simulink model "Counter_condition"  (R2022b)
settings: Solver=VariableStepAuto  StartTime=0.0  StopTime=10.0  RelTol=1e-3
settings Model: Creator=USER  LastModifiedBy=USER

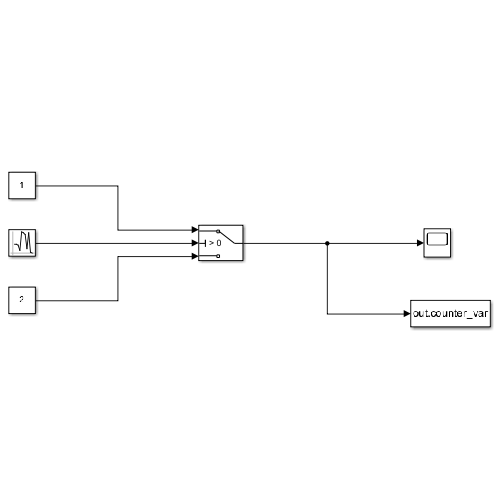
[thumbnail: Simulink's stored preview of the top-level diagram]
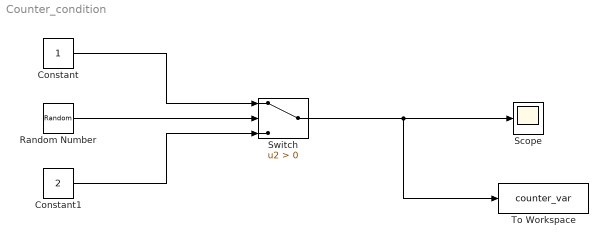
== system Counter_condition ==
  Constant : Constant
  Constant1 : Constant  Value=2
  Random Number : RandomNumber  SampleTime=0.1
  Scope : Scope
  Switch : Switch  Criteria=u2 > Threshold  SaturateOnIntegerOverflow=off  InputSameDT=off
  To Workspace : ToWorkspace  VariableName=counter_var  SaveFormat=Timeseries  SampleTime=-1
  wires:
  Random Number/1 -> Switch/2
  Switch/1 -> To Workspace/1, Scope/1
  Constant/1 -> Switch/1
  Constant1/1 -> Switch/3
